simulink model "untitledPI"  (R2016a)
settings: Solver=VariableStepAuto  StartTime=0.0  StopTime=5  RelTol=1e-3
libraries: powerlib x12, simulink x1, powerlib_extras x1
settings Model: Creator=askit  LastModifiedBy=askit

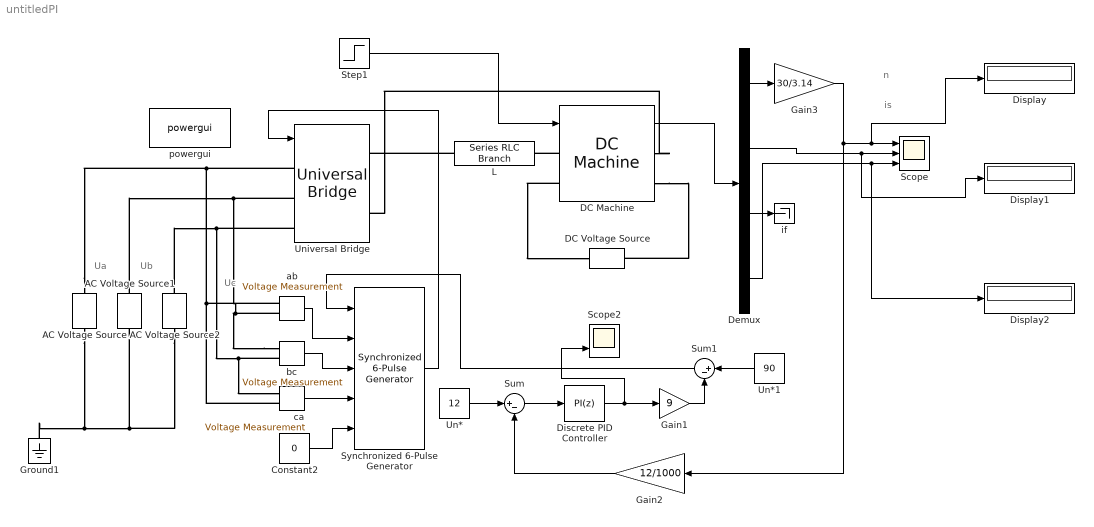
== system untitledPI ==
  note: is
  note: n
  note: Ua
  note: Ub
  note: Uc
  AC Voltage Source : powerlib/Electrical Sources/AC Voltage Source  Amplitude=220  Phase=0  Frequency=50  SampleTime=0  Measurements=None  BusType=swing  Pref=10e3  Qref=0  Qmin=-inf  Qmax=+inf
  AC Voltage Source1 : powerlib/Electrical Sources/AC Voltage Source  Amplitude=220  Phase=240  Frequency=50  SampleTime=0  Measurements=None  BusType=swing  Pref=10e3  Qref=0  Qmin=-inf  Qmax=+inf
  AC Voltage Source2 : powerlib/Electrical Sources/AC Voltage Source  Amplitude=220  Phase=120  Frequency=50  SampleTime=0  Measurements=None  BusType=swing  Pref=10e3  Qref=0  Qmin=-inf  Qmax=+inf
  Constant2 : Constant  Value=0
  DC Machine : powerlib/Machines/DC Machine  PresetModel=No  MechanicalLoad=Torque TL  FieldType=Wound  ShowDetailedParameters=on  MeasurementBus=off  RLa="[ 0.5  0.017]"  RLf="[ 240  120]"  Laf=2.007  MachineConstant=Torque constant (N.m/A)  Ke=1.8  Kt=1.8  J=0.255  Bm=0  Tf=0  w0=1  Ifinit=1  TsPowergui=0  TsBlock=-1
  DC Voltage Source : powerlib/Electrical Sources/DC Voltage Source  Amplitude=220  Measurements=None
  Demux : Demux
  Discrete PID Controller : simulink/Continuous/PID Controller  Controller=PI  TimeDomain=Discrete-time  SampleTime=60e-6  IntegratorMethod=Forward Euler  FilterMethod=Forward Euler  Form=Parallel  UseFilter=on  ControllerParametersSource=internal  P=0.488445657651457  I=12.9670270757228  D=0  N=100  InitialConditionSource=internal  InitialConditionForIntegrator=0  InitialConditionForFilter=0  ExternalReset=none  LimitOutput=on  UpperSaturationLimit=10  LowerSaturationLimit=-10  LinearizeAsGain=off  AntiWindupMode=none  Kb=1  TrackingMode=off  Kt=1  PParamMin=[]  PParamMax=[]  IParamMin=[]  IParamMax=[]  DParamMin=[]  DParamMax=[]  NParamMin=[]  NParamMax=[]  KbParamMin=[]  KbParamMax=[]  KtParamMin=[]  KtParamMax=[]  POutMin=[]  POutMax=[]  IOutMin=[]  IOutMax=[]  DOutMin=[]  DOutMax=[]  NOutMin=[]  NOutMax=[]  KbOutMin=[]  KbOutMax=[]  KtOutMin=[]  KtOutMax=[]  IntegratorOutMin=[]  IntegratorOutMax=[]  FilterOutMin=[]  FilterOutMax=[]  SumOutMin=[]  SumOutMax=[]  SumI1OutMin=[]  SumI1OutMax=[]  SumI2OutMin=[]  SumI2OutMax=[]  SumI3OutMin=[]  SumI3OutMax=[]  SumDOutMin=[]  SumDOutMax=[]  SaturationOutMin=[]  SaturationOutMax=[]  IntegratorContinuousStateAttributes=''  IntegratorStateMustResolveToSignalObject=off  IntegratorRTWStateStorageClass=Auto  FilterContinuousStateAttributes=''  FilterStateMustResolveToSignalObject=off  FilterRTWStateStorageClass=Auto  DifferentiatorICPrevScaledInput=0  DifferentiatorOutMin=[]  DifferentiatorOutMax=[]
  Display : Display
  Display1 : Display
  Display2 : Display
  Gain1 : Gain  Gain=9
  Gain2 : Gain  Gain=12/1000
  Gain3 : Gain  Gain=30/3.14
  Ground1 : powerlib/Elements/Ground  LConnTagsString=a
  L : powerlib/Elements/Series RLC Branch  LConnTagsString=__new0  RConnTagsString=__new0  BranchType=L  Resistance=1  Inductance=1e-3  SetiL0=off  InitialCurrent=0  Capacitance=1e-6  Setx0=off  InitialVoltage=0  Measurements=None
  Scope : Scope  NumInputPorts=3
  Scope2 : Scope  NumInputPorts=2
  Step1 : Step  Time=2  Before=50  After=101.1  SampleTime=0
  Sum : Sum  Inputs=|+-
  Sum1 : Sum  Inputs=|+-
  Synchronized 6-Pulse Generator : powerlib_extras/Control  Blocks/Synchronized 6-Pulse Generator  freq=50  pwidth=5  Double_Pulse=on
  Un* : Constant  Value=12
  Un*1 : Constant  Value=90
  Universal Bridge : powerlib/Power Electronics/Universal Bridge  Arms=3  SnubberResistance=1e5  SnubberCapacitance=inf  Device=Thyristors  Ron=5e-1  Lon=0  ForwardVoltages="[  0  0  ]"  ForwardVoltage=0  GTOparameters=[ 10e-6 , 20e-6 ]  IGBTparameters=[ 1e-6 , 2e-6 ]  Measurements=None  Measurements_2=None  converterType=Rectifier
  ab : powerlib/Measurements/Voltage Measurement  PhasorSimulation=off  OutputType=Complex  PSBequivalent=0
  bc : powerlib/Measurements/Voltage Measurement  PhasorSimulation=off  OutputType=Complex  PSBequivalent=0
  ca : powerlib/Measurements/Voltage Measurement  PhasorSimulation=off  OutputType=Complex  PSBequivalent=0
  if : Terminator
  powergui : powerlib/powergui  Priority=1  SimulationMode=Continuous  SolverType=Tustin/Backward Euler (TBE)  SampleTime=50e-6  frequency=60  SPID=on  DisableSnubberDevices=off  DisableRonSwitches=off  DisableVfSwitches=off  SwTol=0  DisplayEquations=off  Interpol=off  ExternalGateDelay=off  methode=off  Ts=100  FunctionMessages=off  echomessages=off  HookPort=off  EnableUseOfTLC=off  x0status=blocks  frequencyindice=0  Pbase=100e6  ErrMax=1e-4  Iterations=50  UnitsV=kV  UnitsW=MW  buscounter=0  RestoreLinks=warning  ResistiveCurrentMeasurement=off  Frange=[0:2:500]  Ylog=off  Xlog=on  ShowGrid=off  save=off  variable=ZData  structure=0  ZoomFFT=off  StartTime=0.0  cycles=1  DisplayStyle=1  fundamental=60  FreqAxis=off  MaxFrequency=1000  frequencyindicesteady=1  RmsSteady=1  display=off
  wires:
  Discrete PID Controller/1 -> Gain1/1, Scope2/2
  Synchronized 6-Pulse Generator/1 -> Universal Bridge/1
  Sum/1 -> Discrete PID Controller/1
  Un*1/1 -> Sum1/1
  Sum1/1 -> Synchronized 6-Pulse Generator/1
  Un*/1 -> Sum/1
  Constant2/1 -> Synchronized 6-Pulse Generator/5
  bc/1 -> Synchronized 6-Pulse Generator/3
  ab/1 -> Synchronized 6-Pulse Generator/2
  Gain2/1 -> Sum/2
  Demux/2 -> Display1/1, Scope/2
  Demux/3 -> if/1
  Demux/4 -> Display2/1, Scope/3
  DC Machine/1 -> Demux/1
  Gain3/1 -> Display/1, Scope/1, Gain2/1
  ca/1 -> Synchronized 6-Pulse Generator/4
  Demux/1 -> Gain3/1
  Gain1/1 -> Sum1/2
  Step1/1 -> DC Machine/1
  connections:
  AC Voltage Source/RConn1 -- Universal Bridge/LConn1 -- ca/LConn2 -- ab/LConn1
  bc/LConn1 -- ab/LConn2 -- Universal Bridge/LConn2 -- AC Voltage Source1/RConn1
  AC Voltage Source2/RConn1 -- Universal Bridge/LConn3 -- bc/LConn2 -- ca/LConn1
  DC Machine/RConn1 -- Universal Bridge/RConn2
  DC Machine/LConn1 -- L/RConn1
  L/LConn1 -- Universal Bridge/RConn1
  DC Machine/LConn2 -- DC Voltage Source/RConn1
  Ground1/LConn1 -- AC Voltage Source/LConn1 -- AC Voltage Source2/LConn1 -- AC Voltage Source1/LConn1
  DC Machine/RConn2 -- DC Voltage Source/LConn1
